simulink model "EXE1_11"  (R2019b)
settings: Solver=VariableStepAuto  StartTime=0.0  StopTime=0.06  RelTol=1e-3
libraries: powerlib x20, powerlib_meascontrol x4
settings Model: Creator=DELL  LastModifiedBy=DELL

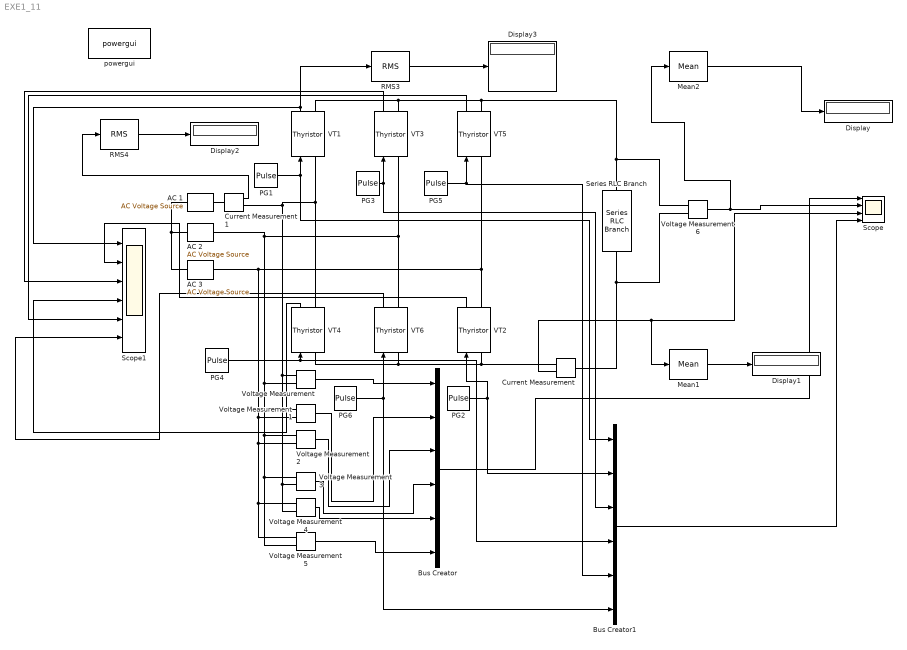
== system EXE1_11 ==
  "AC 1 " : powerlib/Electrical Sources/AC Voltage Source  Amplitude=310  Phase=0  Frequency=50  SampleTime=0  Measurements=None  BusType=swing  Pref=10e3  Qref=0  Qmin=-inf  Qmax=+inf
      settings: SourceProductName=Simscape Electrical
  AC 2 : powerlib/Electrical Sources/AC Voltage Source  Amplitude=310  Phase=-120  Frequency=50  SampleTime=0  Measurements=None  BusType=swing  Pref=10e3  Qref=0  Qmin=-inf  Qmax=+inf
      settings: SourceProductName=Simscape Electrical
  AC 3 : powerlib/Electrical Sources/AC Voltage Source  Amplitude=310  Phase=-240  Frequency=50  SampleTime=0  Measurements=None  BusType=swing  Pref=10e3  Qref=0  Qmin=-inf  Qmax=+inf
      settings: SourceProductName=Simscape Electrical
  Bus Creator : BusCreator  Inputs=6
  Bus Creator1 : BusCreator  Inputs=6
  Current Measurement : powerlib/Measurements/Current Measurement  PhasorSimulation=off  OutputType=Complex  PSBequivalent=0
      settings: SourceProductName=Simscape Electrical
  Current Measurement1 : powerlib/Measurements/Current Measurement  PhasorSimulation=off  OutputType=Complex  PSBequivalent=0
      settings: SourceProductName=Simscape Electrical
  Display{,1..3} (4 alike) : Display
  Mean1 : powerlib_meascontrol/Measurements/Mean  Freq=60  Vinit=0  Ts=0
      settings: SourceProductName=Simscape Electrical
  Mean2 : powerlib_meascontrol/Measurements/Mean  Freq=60  Vinit=0  Ts=0
      settings: SourceProductName=Simscape Electrical
  PG1 : DiscretePulseGenerator  PulseType=Time based  Period=0.02  PulseWidth=20  PhaseDelay=0.0064
  PG2 : DiscretePulseGenerator  PulseType=Time based  Period=0.02  PulseWidth=20  PhaseDelay=0.0097
  PG3 : DiscretePulseGenerator  PulseType=Time based  Period=0.02  PulseWidth=20  PhaseDelay=0.0131
  PG4 : DiscretePulseGenerator  PulseType=Time based  Period=0.02  PulseWidth=20  PhaseDelay=0.0164
  PG5 : DiscretePulseGenerator  PulseType=Time based  Period=0.02  PulseWidth=20  PhaseDelay=0.0197
  PG6 : DiscretePulseGenerator  PulseType=Time based  Period=0.02  PulseWidth=20  PhaseDelay=0.0231
  RMS3 : powerlib_meascontrol/Measurements/RMS  TrueRMS=on  Freq=60  RMSInit=120  Ts=0
      settings: SourceProductName=Simscape Electrical
  RMS4 : powerlib_meascontrol/Measurements/RMS  TrueRMS=on  Freq=60  RMSInit=120  Ts=0
      settings: SourceProductName=Simscape Electrical
  Scope : Scope  NumInputPorts=4
  Scope1 : Scope  NumInputPorts=6
  Series RLC Branch : powerlib/Elements/Series RLC Branch  LConnTagsString=__new0  RConnTagsString=__new0  BranchType=RL  Resistance=1  Inductance=5e-3  SetiL0=off  InitialCurrent=0  Capacitance=0  Setx0=off  InitialVoltage=0  Measurements=None
      settings: SourceProductName=Simscape Electrical
  VT{1..6} (6 alike) : powerlib/Power Electronics/Thyristor  Ron=0.001  Lon=0  Vf=0.8  IC=0  Rs=500  Cs=250e-9  Measurements=on
      settings: SourceProductName=Simscape Electrical
  Voltage Measurement{,1..6} (7 alike) : powerlib/Measurements/Voltage Measurement  PhasorSimulation=off  OutputType=Complex  PSBequivalent=0
      settings: SourceProductName=Simscape Electrical
  powergui : powerlib/powergui  Priority=1  SimulationMode=Continuous  SampleTime=50e-6  frequency=60  Iterations=50  frequencyindice=50  Pbase=100e6  ErrMax=1e-4  UnitsV=kV  UnitsW=MW  buscounter=0  FunctionMessages=off  echomessages=off  EnableUseOfTLC=off  CurrentSourceSwitches=off  DisableSnubberDevices=off  DisableRonSwitches=off  DisableVfSwitches=off  DisplayEquations=off  AutomaticDiscreteSolvers=off  SolverType=Tustin/Backward Euler (TBE)  Interpol=off  ExternalGateDelay=off  methode=off  Ts=100  x0status=blocks  SPID=on  SwTol=0  HookPort=off  NonlinearTolerance=1e-4  nMaxIteration=100  ContinueOnMaxIteration=off  RestoreLinks=warning  ResistiveCurrentMeasurement=off  Frange=[0:2:500]  Ylog=off  Xlog=on  ShowGrid=off  save=off  variable=ZData  structure=0  ZoomFFT=off  StartTime=0.0  cycles=1  DisplayStyle=1  fundamental=60  FreqAxis=off  MaxFrequency=1000  frequencyindicesteady=1  RmsSteady=1  display=off
      settings: SourceProductName=Simscape Electrical
  wires:
  Voltage Measurement/1 -> Bus Creator/1
  Voltage Measurement1/1 -> Bus Creator/2
  Voltage Measurement2/1 -> Bus Creator/3
  Voltage Measurement3/1 -> Bus Creator/4
  Voltage Measurement4/1 -> Bus Creator/5
  Voltage Measurement5/1 -> Bus Creator/6
  Bus Creator/1 -> Scope/1
  PG1/1 -> Bus Creator1/1, VT1/1
  PG2/1 -> Bus Creator1/2, VT2/1
  PG4/1 -> Bus Creator1/4, VT4/1
  PG5/1 -> Bus Creator1/5, VT5/1
  PG6/1 -> Bus Creator1/6, VT6/1
  Voltage Measurement6/1 -> Mean2/1, Scope/2
  Current Measurement/1 -> Mean1/1, Scope/3
  PG3/1 -> VT3/1, Bus Creator1/3
  Bus Creator1/1 -> Scope/4
  Current Measurement1/1 -> RMS4/1
  Mean2/1 -> Display/1
  Mean1/1 -> Display1/1
  VT1/1 -> Scope1/1, RMS3/1
  RMS3/1 -> Display3/1
  RMS4/1 -> Display2/1
  VT2/1 -> Scope1/2
  VT3/1 -> Scope1/3
  VT4/1 -> Scope1/4
  VT5/1 -> Scope1/5
  VT6/1 -> Scope1/6
  connections:
  VT4/RConn1 -- Current Measurement1/RConn1 -- Voltage Measurement4/LConn2 -- Voltage Measurement3/LConn2 -- Voltage Measurement1/LConn1 -- Voltage Measurement/LConn1 -- VT1/LConn1
  VT6/RConn1 -- Voltage Measurement2/LConn1 -- Voltage Measurement5/LConn2 -- Voltage Measurement3/LConn1 -- Voltage Measurement/LConn2 -- AC 2/RConn1 -- VT3/LConn1
  VT2/RConn1 -- Voltage Measurement5/LConn1 -- Voltage Measurement4/LConn1 -- Voltage Measurement2/LConn2 -- Voltage Measurement1/LConn2 -- AC 3/RConn1 -- VT5/LConn1
  VT1/RConn1 -- VT3/RConn1 -- VT5/RConn1 -- Voltage Measurement6/LConn1 -- Series RLC Branch/LConn1
  VT4/LConn1 -- Current Measurement/RConn1 -- VT2/LConn1 -- VT6/LConn1
  Current Measurement/LConn1 -- Voltage Measurement6/LConn2 -- Series RLC Branch/RConn1
  "AC 1 "/LConn1 -- AC 3/LConn1 -- AC 2/LConn1
  Current Measurement1/LConn1 -- "AC 1 "/RConn1
